simulink library "bcm"  (R2021b)
settings: Solver=VariableStepAuto  StartTime=0.0  StopTime=10.0  RelTol=1e-3
undefined symbols (not defined in the file or in its folder): ENUM_ANTITHEFT_ALARM, ENUM_ANTITHEFT_ARM, ENUM_ANTITHEFT_DISARM, ENUM_ANTITHEFT_WAIT, ENUM_GEARPOSNTOCAN_P, ENUM_PDKEYRAWLULOCK_INUNLOCK, ENUM_PDKEYRAWPS_INPS, ENUM_POWERSTA_ON, ENUM_POWERSTA_READY, ENUM_POWERSTA_STANDBY, ENUM_PWRSTASW_ON, ENUM_PWRSTASW_READY, ENUM_VEHICLETYPE_D21, ENUM_VEHICLETYPE_D31F25, ENUM_VEHICLETYPE_D31HAWD, ENUM_VEHICLETYPE_D31HRWD, ENUM_VEHICLETYPE_D31L24, FALSE, KBCM_ACCSwcPrsTmr_s, KBCM_ALMBrightnessDark_enum, KBCM_AmbBlue_enum, KBCM_AmbBreathT_ms, KBCM_AmbGreen_enum, KBCM_AmbMidPple_enum, KBCM_AmbRed_enum, KBCM_AmbTempCtrlEN_flg, KBCM_AmbTempT_s, KBCM_AmbWelModeENWait_s, KBCM_Antitheft_enum_ovrdflg, KBCM_Antitheft_enum_ovrdval, KBCM_APMDoorCtrlSta_flg_ovrdflg, KBCM_APMDoorCtrlSta_flg_ovrdval, KBCM_CmdKeepT_s, KBCM_CSWLightRstDebT_s, KBCM_CSWTurnLPRstT_s, KBCM_DelayTSW_flg, KBCM_DiagDRLOFF_flg, KBCM_DiagFLTC_mA, KBCM_DiagFMHT_s, KBCM_DiagFRTC_mA, KBCM_DiagRLTC_mA, KBCM_DiagRRTC_mA, KBCM_DrAPMRetryTimes_cnt, KBCM_DrOpenWdwOT_s, KBCM_DrOpenWdwReady_s, KBCM_ESSOffT_ms, KBCM_ESSOnT_ms, KBCM_FDCDKCReDetectT_K, KBCM_FDCDKCUSSFilterT_K, KBCM_HandleLampKeepT_s, KBCM_IVIRstHoldT_ms, KBCM_IVIRstTriggerT_ms, KBCM_ONDelayT_ms, KBCM_RAPSAbnFlashOFFT_ms, KBCM_RAPSAbnFlashONT_ms, KBCM_ReDetectT_K, KBCM_RightHandDriveEN_flg, KBCM_RLSLowSpdFilterT_s, KBCM_RmLampKeep_min, KBCM_RmLpKeyInT_s ... (+37)
libraries: simulink x389, $bdroot x11, hcu_lib x2
(part 5 of 13)

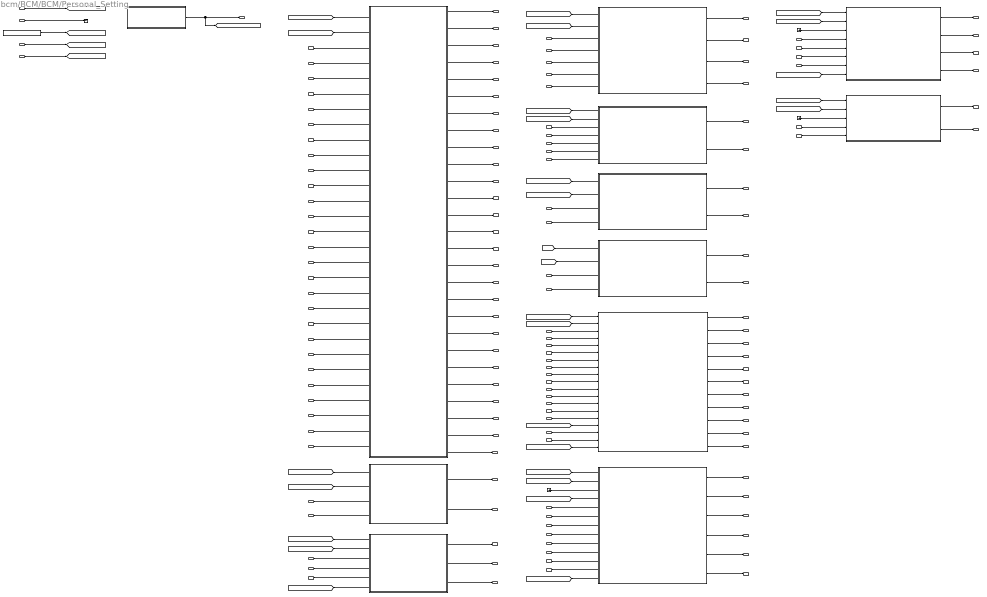
== system bcm/BCM/BCM/Personal_Setting ==
  task_time_s : Inport
  UserNow : Inport  Port=2
  VINP_CANMsgValidIVI1_flg : Inport  Port=3
  VINP_AmbLightSW_flg : Inport  Port=4
  VINP_FlashAmbFunEN_enum : Inport  Port=5
  VINP_AmbLightWlcmLightSW_flg : Inport  Port=6
  VINP_FlashAmbWelEN_enum : Inport  Port=7
  VINP_AmbLightDimInDarkSW_flg : Inport  Port=8
  VINP_FlashAmbDimEN_enum : Inport  Port=9
  VINP_LINKtoDRIVE_flg : Inport  Port=10
  VINP_FlashAmbLinkDriSta_enum : Inport  Port=11
  VINP_AmbLighLowBatAlertSW_flg : Inport  Port=12
  VINP_FlashAmbPwrWarnEN_enum : Inport  Port=13
  VINP_AmbLighSafetyAlertSW_flg : Inport  Port=14
  VINP_FlashAmbODAEN_enum : Inport  Port=15
  VINP_AmbLightColorSet_enum : Inport  Port=16
  VINP_FlashAmbColorSta1_enum : Inport  Port=17
  VINP_FlashAmbColorSta2_enum : Inport  Port=18
  VINP_FlashAmbColorSta3_enum : Inport  Port=19
  VINP_FlashAmbColorSta4_enum : Inport  Port=20
  VINP_FlashAmbColorSta5_enum : Inport  Port=21
  VINP_FlashAmbColorSta7_enum : Inport  Port=22
  VINP_AmbLightBrightnessSet_enum : Inport  Port=23
  VINP_FlashAmbBrightnessSta1_enum : Inport  Port=24
  VINP_FlashAmbBrightnessSta2_enum : Inport  Port=25
  VINP_FlashAmbBrightnessSta3_enum : Inport  Port=26
  VINP_FlashAmbBrightnessSta4_enum : Inport  Port=27
  VINP_FlashAmbBrightnessSta5_enum : Inport  Port=28
  VINP_FlashAmbBrightnessSta7_enum : Inport  Port=29
  VINP_IVIPTGUSStaSW_flg : Inport  Port=30
  VINP_FlashSPTGENFun_enum : Inport  Port=31
  VINP_TurnSwTimeSet_enum : Inport  Port=32
  VINP_FlashTurnSwTimeSetSta123_enum : Inport  Port=33
  VINP_FlashTurnSwTimeSetSta457_enum : Inport  Port=34
  VINP_CANMsgValidIVI2_flg : Inport  Port=35
  VINP_ApproachUnlockSW_flg : Inport  Port=36
  VINP_FlashWalkInUnLkEn_enum : Inport  Port=37
  VINP_WalkawayLockSW_flg : Inport  Port=38
  VINP_FlashWalkOutLkEn_enum : Inport  Port=39
  VINP_RoomLampMode_flg : Inport  Port=40
  VINP_FlashRmLpModeEN_enum : Inport  Port=41
  VINP_SetUnlockSingle_flg : Inport  Port=42
  VINP_FlashLockSettingSta_enum : Inport  Port=43
  VINP_FollowMeSW_flg : Inport  Port=44
  VINP_FlashFollowMeENFun_enum : Inport  Port=45
  VINP_IVIPTGOpenHeight_enum : Inport  Port=46
  VINP_FlashPTGOpenHeight12_enum : Inport  Port=47
  VINP_FlashPTGOpenHeight34_enum : Inport  Port=48
  VINP_FlashPTGOpenHeight57_enum : Inport  Port=49
  VINP_PTGIsSetHeight_flg : Inport  Port=50
  VINP_BPPTGIsSetHeightSta_flg : Inport  Port=51
  VINP_PTGLeftHallPosn_cnt : Inport  Port=52
  VINP_FlashPTGUserHeight1_cnt : Inport  Port=53
  VINP_FlashPTGUserHeight2_cnt : Inport  Port=54
  VINP_FlashPTGUserHeight3_cnt : Inport  Port=55
  VINP_FlashPTGUserHeight4_cnt : Inport  Port=56
  VINP_FlashPTGUserHeight5_cnt : Inport  Port=57
  VINP_FlashPTGUserHeight7_cnt : Inport  Port=58
  VINP_TimeGapLevel_enum : Inport  Port=59
  VINP_FlashACCLevelSta12_enum : Inport  Port=60
  VINP_FlashACCLevelSta34_enum : Inport  Port=61
  VINP_FlashACCLevelSta57_enum : Inport  Port=62
  VINP_SWC2LRightSta_flg : Inport  Port=63
  VINP_SWC2LLeftSta_flg : Inport  Port=64
  VINP_FDCVMCSpdCtrlModeSta_enum : Inport  Port=65
  VINP_ADASACCSta_enum : Inport  Port=66
  VINP_IVIStoppingUnlockSWSta_flg : Inport  Port=67
  VINP_FlashAutoLock_enum : Inport  Port=68
  VINP_IVIDrivingLockSWSta_flg : Inport  Port=69
  VINP_FlashAutoUnlock_enum : Inport  Port=70
  VINP_CANMsgValidBodyZonePS1_flg : Inport  Port=71
  VINP_LeftHallPos_cnt : Inport  Port=72
  VINP_VehicleType_enum : Inport  Port=73
  VINP_SWC2RCustomizeSta_flg : Inport  Port=74
  VINP_IVISWCRUndefinedSta_enum : Inport  Port=75
  VINP_HMIAutoInterLightCmd_flg : Inport  Port=76
  VINP_IVICLWinLockDrSW_flg : Inport  Port=77
  VINP_FlashCLWinLockDrSta_enum : Inport  Port=78
  VINP_IVICarWashModeCmd_flg : Inport  Port=79
  ACC : Subsystem
  AmbLight : Subsystem
  Autolock : Subsystem
  Constant : Constant  Value=KBCM_UserFix_enum
  DKC_Lock_Setting : Subsystem
  FlasherSignal : Subsystem
  FollowMeHome : Subsystem
  Ground : Ground
  Ground1 : Ground
  Ground4 : Ground
  LockSetting : Subsystem
  PTG : Subsystem
  RoomLamp : Subsystem
  SPTG : Subsystem
  System_Loadbar : Subsystem
  Terminator : Terminator
  Window : Subsystem
  Loadbar : Outport
  VBCM_UserNow_enum : Outport  Port=2
  FDC_BCM_AmbFunEN_Sta : Outport  Port=3
  VBCM_AmbFunENMem_enum : Outport  Port=4
  FDC_BCM_AmbWelEN_Sta : Outport  Port=5
  VBCM_AmbWelENMem_enum : Outport  Port=6
  FDC_BCM_AmbDimEN_Sta : Outport  Port=7
  VBCM_AmbDimENMem_enum : Outport  Port=8
  FDC_BCM_AmbLinkDriSta_Sta : Outport  Port=9
  VBCM_AmbLinkDriStaMem_enum : Outport  Port=10
  FDC_BCM_AmbPwrWarnEN_Sta : Outport  Port=11
  VBCM_AmbPwrWarnENMem_enum : Outport  Port=12
  FDC_BCM_AmbODAEN_Sta : Outport  Port=13
  VBCM_AmbODAENMem_enum : Outport  Port=14
  FDC_BCM_AmbColorSta_Sta : Outport  Port=15
  VBCM_AmbColorSta1_enum : Outport  Port=16
  VBCM_AmbColorSta2_enum : Outport  Port=17
  VBCM_AmbColorSta3_enum : Outport  Port=18
  VBCM_AmbColorSta4_enum : Outport  Port=19
  VBCM_AmbColorSta5_enum : Outport  Port=20
  VBCM_AmbColorSta7_enum : Outport  Port=21
  FDC_BCM_AmbBrightSta_Sta : Outport  Port=22
  VBCM_AmbBrightnessSta1_enum : Outport  Port=23
  VBCM_AmbBrightnessSta2_enum : Outport  Port=24
  VBCM_AmbBrightnessSta3_enum : Outport  Port=25
  VBCM_AmbBrightnessSta4_enum : Outport  Port=26
  VBCM_AmbBrightnessSta5_enum : Outport  Port=27
  VBCM_AmbBrightnessSta7_enum : Outport  Port=28
  VBCM_SPTGENFun_flg : Outport  Port=29
  VBCM_SPTGENFunMem_enum : Outport  Port=30
  VBCM_TurnSwTSetSta_enum : Outport  Port=31
  VBCM_TurnSwTimeSetSta123_enum : Outport  Port=32
  VBCM_TurnSwTimeSetSta457_enum : Outport  Port=33
  FDC_BCM_WalkInUnLkEnFun_Sta : Outport  Port=34
  VBCM_WalkInUnLkEnMem_enum : Outport  Port=35
  FDC_BCM_WalkOutLkEnFun_Sta : Outport  Port=36
  VBCM_WalkOutLkEnMem_enum : Outport  Port=37
  FDC_BCM_RmLpModeENFun_Sta : Outport  Port=38
  VBCM_RmLpModeENMem_enum : Outport  Port=39
  VBCM_LockSetting_flg : Outport  Port=40
  VBCM_LockSettingStaMem_enum : Outport  Port=41
  FDC_BCM_FollowMeENFun_Sta : Outport  Port=42
  VBCM_FollowMeENMem_enum : Outport  Port=43
  VBCM_PTGOpenHeightSta_enum : Outport  Port=44
  VBCM_UserHeightSet_cnt : Outport  Port=45
  VBCM_PTGUserHeight1_cnt : Outport  Port=46
  VBCM_PTGUserHeight2_cnt : Outport  Port=47
  VBCM_PTGUserHeight3_cnt : Outport  Port=48
  VBCM_PTGUserHeight4_cnt : Outport  Port=49
  VBCM_PTGUserHeight5_cnt : Outport  Port=50
  VBCM_PTGUserHeight7_cnt : Outport  Port=51
  VBCM_PTGOpenHeight12_enum : Outport  Port=52
  VBCM_PTGOpenHeight34_enum : Outport  Port=53
  VBCM_PTGOpenHeight57_enum : Outport  Port=54
  VBCM_TimeGapLevelSta_enum : Outport  Port=55
  VBCM_ACCLevelMem12_enum : Outport  Port=56
  VBCM_ACCLevelMem34_enum : Outport  Port=57
  VBCM_ACCLevelMem57_enum : Outport  Port=58
  VBCM_LRightStaCmd_flg : Outport  Port=59
  VBCM_LLeftStaCmd_flg : Outport  Port=60
  VBCM_AutoLockSta_flg : Outport  Port=61
  VBCM_AutoLockMem_enum : Outport  Port=62
  VBCM_AutoUnlockSta_flg : Outport  Port=63
  VBCM_AutoUnlockMem_enum : Outport  Port=64
  VBCM_CLWinLockDrSta_flg : Outport  Port=65
  VBCM_CLWinLockDrStaMem_enum : Outport  Port=66
  wires:
  VINP_FlashAmbFunEN_enum/1 -> AmbLight/5(VINP_FlashAmbFunEN_enum)
  VINP_FlashAmbBrightnessSta3_enum/1 -> AmbLight/26(VINP_FlashAmbBrightnessSta3_enum)
  VINP_FlashAmbBrightnessSta7_enum/1 -> AmbLight/29(VINP_FlashAmbBrightnessSta7_enum)
  VINP_FlashAmbColorSta7_enum/1 -> AmbLight/22(VINP_FlashAmbColorSta7_enum)
  VINP_FlashAmbColorSta5_enum/1 -> AmbLight/21(VINP_FlashAmbColorSta5_enum)
  VINP_FlashAmbColorSta1_enum/1 -> AmbLight/17(VINP_FlashAmbColorSta1_enum)
  VINP_FlashAmbDimEN_enum/1 -> AmbLight/9(VINP_FlashAmbDimEN_enum)
  VINP_AmbLightSW_flg/1 -> AmbLight/4(VINP_AmbLightSW_flg)
  VINP_FlashAmbColorSta3_enum/1 -> AmbLight/19(VINP_FlashAmbColorSta3_enum)
  VINP_FlashAmbColorSta4_enum/1 -> AmbLight/20(VINP_FlashAmbColorSta4_enum)
  VINP_FlashAmbODAEN_enum/1 -> AmbLight/15(VINP_FlashAmbODAEN_enum)
  VINP_AmbLightWlcmLightSW_flg/1 -> AmbLight/6(VINP_AmbLightWlcmLightSW_flg)
  AmbLight/4(FDC_BCM_AmbWelEN_Sta) -> FDC_BCM_AmbWelEN_Sta/1
  VINP_AmbLighLowBatAlertSW_flg/1 -> AmbLight/12(VINP_AmbLighLowBatAlertSW_flg)
  AmbLight/14(FDC_BCM_AmbColorSta_Sta) -> FDC_BCM_AmbColorSta_Sta/1
  AmbLight/10(FDC_BCM_AmbPwrWarnEN_Sta) -> FDC_BCM_AmbPwrWarnEN_Sta/1
  VINP_AmbLightBrightnessSet_enum/1 -> AmbLight/23(VINP_AmbLightBrightnessSet_enum)
  VINP_AmbLighSafetyAlertSW_flg/1 -> AmbLight/14(VINP_AmbLighSafetyAlertSW_flg)
  AmbLight/2(FDC_BCM_AmbFunEN_Sta) -> FDC_BCM_AmbFunEN_Sta/1
  AmbLight/6(FDC_BCM_AmbDimEN_Sta) -> FDC_BCM_AmbDimEN_Sta/1
  AmbLight/8(FDC_BCM_AmbLinkDriSta_Sta) -> FDC_BCM_AmbLinkDriSta_Sta/1
  VINP_LINKtoDRIVE_flg/1 -> AmbLight/10(VINP_LINKtoDRIVE_flg)
  VINP_FlashAmbBrightnessSta2_enum/1 -> AmbLight/25(VINP_FlashAmbBrightnessSta2_enum)
  VINP_FlashAmbColorSta2_enum/1 -> AmbLight/18(VINP_FlashAmbColorSta2_enum)
  VINP_AmbLightDimInDarkSW_flg/1 -> AmbLight/8(VINP_AmbLightDimInDarkSW_flg)
  VINP_FlashAmbLinkDriSta_enum/1 -> AmbLight/11(VINP_FlashAmbLinkDriSta_enum)
  VINP_AmbLightColorSet_enum/1 -> AmbLight/16(VINP_AmbLightColorSet_enum)
  VINP_FlashAmbBrightnessSta4_enum/1 -> AmbLight/27(VINP_FlashAmbBrightnessSta4_enum)
  VINP_FlashAmbPwrWarnEN_enum/1 -> AmbLight/13(VINP_FlashAmbPwrWarnEN_enum)
  [Loadbar] -> AmbLight/2(Loadbar)
  VINP_FlashAmbBrightnessSta5_enum/1 -> AmbLight/28(VINP_FlashAmbBrightnessSta5_enum)
  VINP_FlashAmbBrightnessSta1_enum/1 -> AmbLight/24(VINP_FlashAmbBrightnessSta1_enum)
  AmbLight/21(FDC_BCM_AmbBrightSta_Sta) -> FDC_BCM_AmbBrightSta_Sta/1
  AmbLight/12(FDC_BCM_AmbODAEN_Sta) -> FDC_BCM_AmbODAEN_Sta/1
  VINP_FlashAmbWelEN_enum/1 -> AmbLight/7(VINP_FlashAmbWelEN_enum)
  System_Loadbar/1(Loadbar) -> [Loadbar], Loadbar/1
  AmbLight/3(VBCM_AmbFunENMem_enum) -> VBCM_AmbFunENMem_enum/1
  AmbLight/5(VBCM_AmbWelENMem_enum) -> VBCM_AmbWelENMem_enum/1
  AmbLight/7(VBCM_AmbDimENMem_enum) -> VBCM_AmbDimENMem_enum/1
  AmbLight/9(VBCM_AmbLinkDriStaMem_enum) -> VBCM_AmbLinkDriStaMem_enum/1
  AmbLight/11(VBCM_AmbPwrWarnENMem_enum) -> VBCM_AmbPwrWarnENMem_enum/1
  AmbLight/13(VBCM_AmbODAENMem_enum) -> VBCM_AmbODAENMem_enum/1
  AmbLight/15(VBCM_AmbColorSta1_enum) -> VBCM_AmbColorSta1_enum/1
  AmbLight/16(VBCM_AmbColorSta2_enum) -> VBCM_AmbColorSta2_enum/1
  AmbLight/17(VBCM_AmbColorSta3_enum) -> VBCM_AmbColorSta3_enum/1
  AmbLight/18(VBCM_AmbColorSta4_enum) -> VBCM_AmbColorSta4_enum/1
  AmbLight/19(VBCM_AmbColorSta5_enum) -> VBCM_AmbColorSta5_enum/1
  AmbLight/20(VBCM_AmbColorSta7_enum) -> VBCM_AmbColorSta7_enum/1
  AmbLight/22(VBCM_AmbBrightnessSta1_enum) -> VBCM_AmbBrightnessSta1_enum/1
  AmbLight/23(VBCM_AmbBrightnessSta2_enum) -> VBCM_AmbBrightnessSta2_enum/1
  AmbLight/24(VBCM_AmbBrightnessSta3_enum) -> VBCM_AmbBrightnessSta3_enum/1
  AmbLight/25(VBCM_AmbBrightnessSta4_enum) -> VBCM_AmbBrightnessSta4_enum/1
  AmbLight/26(VBCM_AmbBrightnessSta5_enum) -> VBCM_AmbBrightnessSta5_enum/1
  AmbLight/27(VBCM_AmbBrightnessSta7_enum) -> VBCM_AmbBrightnessSta7_enum/1
  VINP_CANMsgValidIVI1_flg/1 -> AmbLight/3(VINP_CANMsgValidIVI1_flg)
  AmbLight/1(VBCM_UserNow_enum) -> VBCM_UserNow_enum/1
  SPTG/1(FDC_SPTG_SPTGENFun_Sta) -> VBCM_SPTGENFun_flg/1  "VBCM_SPTGENFun_flg"
  SPTG/2(VBCM_SPTGENFunMem_enum) -> VBCM_SPTGENFunMem_enum/1  "VBCM_SPTGENFunMem_enum"
  [UserNow] -> AmbLight/1(UserNow)
  [UserNow] -> SPTG/1(UserNow)
  UserNow/1 -> Terminator/1
  [Loadbar] -> SPTG/2(Loadbar)
  VINP_IVIPTGUSStaSW_flg/1 -> SPTG/3(VINP_IVIPTGUSStaSW_flg)
  VINP_FlashSPTGENFun_enum/1 -> SPTG/4(VINP_FlashSPTGENFun_enum)
  [UserNow] -> FlasherSignal/1(UserNow)
  [Loadbar] -> FlasherSignal/2(Loadbar)
  FlasherSignal/1(FDC_BCM_TurnSwTSetSta_Sta) -> VBCM_TurnSwTSetSta_enum/1  "FDC_BCM_TurnSwTSetSta_Sta"
  FlasherSignal/2(VBCM_TurnSwTimeSetSta123_enum) -> VBCM_TurnSwTimeSetSta123_enum/1  "VBCM_TurnSwTimeSetSta123_enum"
  FlasherSignal/3(VBCM_TurnSwTimeSetSta457_enum) -> VBCM_TurnSwTimeSetSta457_enum/1  "VBCM_TurnSwTimeSetSta457_enum"
  VINP_TurnSwTimeSet_enum/1 -> FlasherSignal/3(VINP_TurnSwTimeSet_enum)
  VINP_FlashTurnSwTimeSetSta457_enum/1 -> FlasherSignal/5(VINP_FlashTurnSwTimeSetSta457_enum)
  VINP_FlashTurnSwTimeSetSta123_enum/1 -> FlasherSignal/4(VINP_FlashTurnSwTimeSetSta123_enum)
  Constant/1 -> [UserNow]
  [Loadbar] -> DKC_Lock_Setting/2(Loadbar)
  [UserNow] -> DKC_Lock_Setting/1(UserNow)
  VINP_ApproachUnlockSW_flg/1 -> DKC_Lock_Setting/3(VINP_ApproachUnlockSW_flg)
  VINP_FlashWalkInUnLkEn_enum/1 -> DKC_Lock_Setting/4(VINP_FlashWalkInUnLkEn_enum)
  VINP_WalkawayLockSW_flg/1 -> DKC_Lock_Setting/6(VINP_WalkawayLockSW_flg)
  VINP_FlashWalkOutLkEn_enum/1 -> DKC_Lock_Setting/7(VINP_FlashWalkOutLkEn_enum)
  DKC_Lock_Setting/1(FDC_BCM_WalkInUnLkEnFun_Sta) -> FDC_BCM_WalkInUnLkEnFun_Sta/1
  DKC_Lock_Setting/2(VBCM_WalkInUnLkEnMem_enum) -> VBCM_WalkInUnLkEnMem_enum/1
  DKC_Lock_Setting/3(FDC_BCM_WalkOutLkEnFun_Sta) -> FDC_BCM_WalkOutLkEnFun_Sta/1
  DKC_Lock_Setting/4(VBCM_WalkOutLkEnMem_enum) -> VBCM_WalkOutLkEnMem_enum/1
  [Loadbar] -> RoomLamp/2(Loadbar)
  [UserNow] -> RoomLamp/1(UserNow)
  VINP_RoomLampMode_flg/1 -> RoomLamp/3(VINP_RoomLampMode_flg)
  VINP_FlashRmLpModeEN_enum/1 -> RoomLamp/4(VINP_FlashRmLpModeEN_enum)
  RoomLamp/1(FDC_BCM_RmLpModeENFun_Sta) -> FDC_BCM_RmLpModeENFun_Sta/1
  RoomLamp/2(VBCM_RmLpModeENMem_enum) -> VBCM_RmLpModeENMem_enum/1
  LockSetting/2(VBCM_LockSettingStaMem_enum) -> VBCM_LockSettingStaMem_enum/1
  LockSetting/1(VBCM_LockSetting_flg) -> VBCM_LockSetting_flg/1
  VINP_FlashLockSettingSta_enum/1 -> LockSetting/4(VINP_FlashLockSettingSta_enum)
  VINP_SetUnlockSingle_flg/1 -> LockSetting/3(VINP_SetUnlockSingle_flg)
  [UserNow] -> LockSetting/1(UserNow)
  [Loadbar] -> LockSetting/2(Loadbar)
  [Loadbar] -> FollowMeHome/2(Loadbar)
  [UserNow] -> FollowMeHome/1(UserNow)
  VINP_FollowMeSW_flg/1 -> FollowMeHome/3(VINP_FollowMeSW_flg)
  VINP_FlashFollowMeENFun_enum/1 -> FollowMeHome/4(VINP_FlashFollowMeENFun_enum)
  FollowMeHome/1(FDC_BCM_FollowMeENFun_Sta) -> FDC_BCM_FollowMeENFun_Sta/1
  FollowMeHome/2(VBCM_FollowMeENMem_enum) -> VBCM_FollowMeENMem_enum/1
  PTG/2(VBCM_UserHeightSet_cnt) -> VBCM_UserHeightSet_cnt/1
  PTG/1(VBCM_PTGOpenHeightSta_enum) -> VBCM_PTGOpenHeightSta_enum/1
  PTG/7(VBCM_PTGUserHeight5_cnt) -> VBCM_PTGUserHeight5_cnt/1
  PTG/8(VBCM_PTGUserHeight7_cnt) -> VBCM_PTGUserHeight7_cnt/1
  PTG/4(VBCM_PTGUserHeight2_cnt) -> VBCM_PTGUserHeight2_cnt/1
  PTG/5(VBCM_PTGUserHeight3_cnt) -> VBCM_PTGUserHeight3_cnt/1
  PTG/6(VBCM_PTGUserHeight4_cnt) -> VBCM_PTGUserHeight4_cnt/1
  PTG/3(VBCM_PTGUserHeight1_cnt) -> VBCM_PTGUserHeight1_cnt/1
  VINP_CANMsgValidIVI2_flg/1 -> [VINP_CANMsgValidIVI2_flg]
  [VINP_CANMsgValidIVI2_flg] -> FlasherSignal/6(VINP_CANMsgValidIVI2_flg)
  [VINP_CANMsgValidIVI2_flg] -> PTG/16(VINP_CANMsgValidIVI2_flg)
  [Loadbar] -> PTG/2(Loadbar)
  [UserNow] -> PTG/1(UserNow)
  VINP_IVIPTGOpenHeight_enum/1 -> PTG/3(VINP_IVIPTGOpenHeight_enum)
  VINP_FlashPTGOpenHeight12_enum/1 -> PTG/4(VINP_FlashPTGOpenHeight12_enum)
  VINP_BPPTGIsSetHeightSta_flg/1 -> PTG/8(VINP_BPPTGIsSetHeightSta_flg)
  VINP_FlashPTGOpenHeight34_enum/1 -> PTG/5(VINP_FlashPTGOpenHeight34_enum)
  VINP_FlashPTGOpenHeight57_enum/1 -> PTG/6(VINP_FlashPTGOpenHeight57_enum)
  VINP_PTGLeftHallPosn_cnt/1 -> PTG/9(VINP_PTGLeftHallPosn_cnt)
  VINP_FlashPTGUserHeight1_cnt/1 -> PTG/10(VINP_FlashPTGUserHeight1_cnt)
  VINP_FlashPTGUserHeight2_cnt/1 -> PTG/11(VINP_FlashPTGUserHeight2_cnt)
  VINP_FlashPTGUserHeight3_cnt/1 -> PTG/12(VINP_FlashPTGUserHeight3_cnt)
  VINP_FlashPTGUserHeight4_cnt/1 -> PTG/13(VINP_FlashPTGUserHeight4_cnt)
  VINP_FlashPTGUserHeight5_cnt/1 -> PTG/14(VINP_FlashPTGUserHeight5_cnt)
  VINP_FlashPTGUserHeight7_cnt/1 -> PTG/15(VINP_FlashPTGUserHeight7_cnt)
  PTG/9(VBCM_PTGOpenHeight12_enum) -> VBCM_PTGOpenHeight12_enum/1
  PTG/10(VBCM_PTGOpenHeight34_enum) -> VBCM_PTGOpenHeight34_enum/1
  PTG/11(VBCM_PTGOpenHeight57_enum) -> VBCM_PTGOpenHeight57_enum/1
  VINP_PTGIsSetHeight_flg/1 -> PTG/7(VINP_PTGIsSetHeight_flg)
  VINP_SWC2LRightSta_flg/1 -> ACC/9(VINP_SWC2LRightSta_flg)
  ACC/3(VBCM_ACCLevelMem34_enum) -> VBCM_ACCLevelMem34_enum/1
  ACC/4(VBCM_ACCLevelMem57_enum) -> VBCM_ACCLevelMem57_enum/1
  [UserNow] -> ACC/1(UserNow)
  ACC/5(VBCM_LRightStaCmd_flg) -> VBCM_LRightStaCmd_flg/1
  VINP_FDCVMCSpdCtrlModeSta_enum/1 -> ACC/11(VINP_FDCVMCSpdCtrlModeSta_enum)
  ACC/1(VBCM_TimeGapLevelSta_enum) -> VBCM_TimeGapLevelSta_enum/1
  VINP_ADASACCSta_enum/1 -> ACC/12(VINP_ADASACCSta_enum)
  ACC/6(VBCM_LLeftStaCmd_flg) -> VBCM_LLeftStaCmd_flg/1
  ACC/2(VBCM_ACCLevelMem12_enum) -> VBCM_ACCLevelMem12_enum/1
  VINP_FlashACCLevelSta12_enum/1 -> ACC/6(VINP_FlashACCLevelSta12_enum)
  VINP_SWC2LLeftSta_flg/1 -> ACC/10(VINP_SWC2LLeftSta_flg)
  VINP_FlashACCLevelSta57_enum/1 -> ACC/8(VINP_FlashACCLevelSta57_enum)
  VINP_FlashACCLevelSta34_enum/1 -> ACC/7(VINP_FlashACCLevelSta34_enum)
  [task_time_s] -> ACC/4(task_time_s)
  VINP_TimeGapLevel_enum/1 -> ACC/5(VINP_TimeGapLevel_enum)
  Ground/1 -> ACC/3(UpdateReq)
  [Loadbar] -> ACC/2(Loadbar)
  task_time_s/1 -> [task_time_s]
  VINP_IVIStoppingUnlockSWSta_flg/1 -> Autolock/4(VINP_IVIStoppingUnlockSWSta_flg)
  Autolock/3(VBCM_AutoUnlockSta_flg) -> VBCM_AutoUnlockSta_flg/1
  Autolock/4(VBCM_AutoUnlockMem_enum) -> VBCM_AutoUnlockMem_enum/1
  Ground1/1 -> Autolock/3(VBCM_SettingUpdateReq_enum)
  Autolock/2(VBCM_AutoLockMem_enum) -> VBCM_AutoLockMem_enum/1
  VINP_FlashAutoUnlock_enum/1 -> Autolock/7(VINP_FlashAutoUnlock_enum)
  Autolock/1(VBCM_AutoLockSta_flg) -> VBCM_AutoLockSta_flg/1
  VINP_IVIDrivingLockSWSta_flg/1 -> Autolock/6(VINP_IVIDrivingLockSWSta_flg)
  [UserNow] -> Autolock/1(UserNow)
  VINP_FlashAutoLock_enum/1 -> Autolock/5(VINP_FlashAutoLock_enum)
  [Loadbar] -> Autolock/2(Loadbar)
  VINP_CANMsgValidBodyZonePS1_flg/1 -> PTG/17(VINP_CANMsgValidBodyZonePS1_flg)
  VINP_LeftHallPos_cnt/1 -> PTG/18(VINP_LeftHallPos_cnt)
  VINP_VehicleType_enum/1 -> [VINP_VehicleType_enum]
  [VINP_VehicleType_enum] -> ACC/13(VINP_VehicleType_enum)
  [VINP_VehicleType_enum] -> PTG/19(VINP_VehicleType_enum)
  [VINP_VehicleType_enum] -> Autolock/8(VINP_VehicleType_enum)
  VINP_SWC2RCustomizeSta_flg/1 -> RoomLamp/5(VINP_SWC2RCustomizeSta_flg)
  VINP_IVISWCRUndefinedSta_enum/1 -> RoomLamp/6(VINP_IVISWCRUndefinedSta_enum)
  VINP_HMIAutoInterLightCmd_flg/1 -> RoomLamp/7(HMI_AutoInterLight_Cmd)
  Window/1(VBCM_CLWinLockDrSta_flg) -> VBCM_CLWinLockDrSta_flg/1
  Window/2(VBCM_CLWinLockDrStaMem_enum) -> VBCM_CLWinLockDrStaMem_enum/1
  [Loadbar] -> Window/2(Loadbar)
  [UserNow] -> Window/1(UserNow)
  VINP_IVICLWinLockDrSW_flg/1 -> Window/4(VINP_IVICLWinLockDrSW_flg)
  VINP_FlashCLWinLockDrSta_enum/1 -> Window/5(VINP_FlashCLWinLockDrSta_enum)
  Ground4/1 -> Window/3(UpdateReq)
  VINP_IVICarWashModeCmd_flg/1 -> DKC_Lock_Setting/5(VINP_IVICarWashModeCmd_flg)

== system bcm/BCM/BCM/PowerMirror ==
  VPMM_PwrSta_enum : Inport
  VINP_MIRRORFOLDSW_flg : Inport  Port=2
  VINP_VehSpeed_kph : Inport  Port=3
  VBCM_ATActCtrl_enum : Inport  Port=4
  VINP_ReOutsideMirror_enum : Inport  Port=5
  EEP_MFSWTri_flg : Inport  Port=6
  EEP_MirrorFlodPos : Inport  Port=7
  VINP_APSStaSystem_enum : Inport  Port=8
  VINP_IVICarWashModeCmd_flg : Inport  Port=9
  VINP_IVIMirrorFoldedSWSta_flg : Inport  Port=10
  VINP_DKCParkingModeCmd_enum : Inport  Port=11
  AND : Logic  AllPortsSameDT=off  OutDataTypeStr=boolean
  Chart : Stateflow chart  TreatAsAtomicUnit=on
  Compare To Constant : simulink/Logic and Bit Operations/Compare To Constant  relop===  const=0  OutDataTypeStr=boolean
  Compare To Constant1 : simulink/Logic and Bit Operations/Compare To Constant  relop===  const=1  OutDataTypeStr=boolean
  Detect Increase : simulink/Logic and Bit Operations/Detect Increase  vinit=0.0  OutDataTypeStr=boolean
  Unit Delay : UnitDelay  SampleTime=-1  HasFrameUpgradeWarning=on
  VBCM_MirrorCtrl_enum : Outport
  MFSWTri : Outport  Port=2
  MirrorFlodPos : Outport  Port=3
  wires:
  VPMM_PwrSta_enum/1 -> Chart/1(PwrSta)
  VINP_MIRRORFOLDSW_flg/1 -> Chart/2(MirrorFoldSw)
  Chart/1(MirrorCtrl) -> VBCM_MirrorCtrl_enum/1  "VBCM_MirrorCtrl_enum"
  VBCM_ATActCtrl_enum/1 -> Chart/4(ATActCtrl)
  VINP_VehSpeed_kph/1 -> Chart/3(VehSpeed)
  VINP_ReOutsideMirror_enum/1 -> Chart/5(VINP_ReOutsideMirror_enum)
  EEP_MFSWTri_flg/1 -> Chart/6(EEP_MFSWTri_flg)
  EEP_MirrorFlodPos/1 -> Chart/7(EEP_MirrorFlodPos)
  Chart/2(MFSWTri) -> MFSWTri/1  "VBCM_MFSWTri_flg"
  Chart/3(MirrorFlodPos) -> MirrorFlodPos/1  "VBCM_MirrorFlodPos_flg"
  VINP_APSStaSystem_enum/1 -> Chart/8(APS_Sta_System)
  VINP_IVICarWashModeCmd_flg/1 -> Chart/9(IVICarWashModeCmd)
  VINP_IVIMirrorFoldedSWSta_flg/1 -> Detect Increase/1
  Detect Increase/1 -> Chart/10(IVIMirrorFoldedReq)
  AND/1 -> Chart/11(VBCM_RAPSActivate_flg)
  Compare To Constant/1 -> AND/1
  Compare To Constant1/1 -> AND/2
  Unit Delay/1 -> Compare To Constant/1
  VINP_DKCParkingModeCmd_enum/1 -> Compare To Constant1/1, Unit Delay/1

== system bcm/BCM/BCM/RearDefogger ==
  VPMM_PwrSta_enum : Inport
  VINP_RRDefSta_flg : Inport  Port=2
  VINP_IVIRRDefReq_flg : Inport  Port=3
  Chart : Stateflow chart  TreatAsAtomicUnit=on
  VBCM_MirrorDefog_flg : Outport
  VBCM_RrDefog_flg : Outport  Port=2
  wires:
  Chart/1(MirrorDefog) -> VBCM_MirrorDefog_flg/1  "VBCM_MirrorDefog_flg"
  VINP_IVIRRDefReq_flg/1 -> Chart/3(IVI_RR_Def_Req)
  VPMM_PwrSta_enum/1 -> Chart/1(PwrSta)
  Chart/2(RearDefog) -> VBCM_RrDefog_flg/1  "VBCM_RrDefog_flg"
  VINP_RRDefSta_flg/1 -> Chart/2(RR_Def_Sta)

== system bcm/BCM/BCM/RoomLamp ==
  task_time_s : Inport
  VPMM_PwrSta_enum : Inport  Port=2
  VBCM_BCMDoorLockSta_flg : Inport  Port=3
  VBCM_AllDoorSW_flg : Inport  Port=4
  VBCM_AntitheftSta_enum : Inport  Port=5
  VINP_DrDoorSW_flg : Inport  Port=6
  VINP_PsDoorSW_flg : Inport  Port=7
  VINP_RLDoorSW_flg : Inport  Port=8
  VINP_RRDoorSW_flg : Inport  Port=9
  FDC_BCM_RmLpModeENFun_Sta : Inport  Port=10
  VINP_TailgateSW_flg : Inport  Port=11
  KBCM_RmLampKeep_min : Inport  Port=12
  VINP_PDKeyAreaLockUnlock_enum : Inport  Port=13
  VINP_PDKeyAreaPS_enum : Inport  Port=14
  KBCM_RmLpKeyInT_s : Inport  Port=15
  KBCM_RmLpKeyMissT_s : Inport  Port=16
  AND{,1..4} (5 alike) : Logic  AllPortsSameDT=off  OutDataTypeStr=boolean
  Chart : Stateflow chart  TreatAsAtomicUnit=on
      settings: PortSchema="{\"entries\":[{\"content\":{\"sides\":[{\"content\":{\"connectorIds\":[\"In1\",\"In2\",\"In3\",\"In4\",\"In5\",\"In6\",\"In7\",\"In10\",\"In11\",\"In12\",\"In13\",\"In9\",\"In8\"]},\"type\":\"ConnectorPlacement.EquallySpacedRectSide\",\"uuid\":\"6d4ef6e4-d310-4573-8670-c3ce7ffc5586\"},{\"content\":{\"connectorIds\":[\"Out1\",\"Out2\",\"Out3\"],\"side\":\"RIGHT\"},\"type\":\"ConnectorPlacement.EquallySpacedRectSide\",\"uuid\":\"4b29c1e1-9016-4f15-a64e-722acfc91947\"},{\"content\":{\"connectorIds\":[],\"side\":\"TOP\"},\"type\":\"ConnectorPlacement.EquallySpacedRectSide\",\"uuid\":\"c4982b23-9105-4f8b-8d41-99f0f59e85fc\"}]},\"type\":\"ConnectorPlacement.EquallySpacedConnector\",\"uuid\":\"68c6e652-9227-465e-b41e-a009e64da19a\"}],\"packageUris\":[\"http://schema.mathworks.com/mf0/Connector/R2020b\"],\"version\":\"1.0\"}"
  Constant{,1..4} (5 alike) : Constant  OutDataTypeStr=uint8
  Detect Increase{,1..4} (5 alike) : simulink/Logic and Bit Operations/Detect Increase  vinit=0.0  OutDataTypeStr=boolean
  Divide : Product  Inputs=*/
  Gain : Gain  Gain=MIN2SEC
  OR : Logic  Operator=OR  Inputs=5  AllPortsSameDT=off  OutDataTypeStr=boolean
  Terminator : Terminator
  Unit Delay{1..5} (5 alike) : UnitDelay  SampleTime=-1  HasFrameUpgradeWarning=on
  VBCM_RoomLampH_flg : Outport
  VBCM_RoomLampL_flg : Outport  Port=2
  wires:
  VBCM_BCMDoorLockSta_flg/1 -> Chart/3(DrLockSW)
  Chart/2(RoomLampL) -> VBCM_RoomLampL_flg/1  "VBCM_RoomLampL_flg"
  VPMM_PwrSta_enum/1 -> Chart/2(PwrSta)
  VBCM_AllDoorSW_flg/1 -> Chart/4(AllDoorSW)
  Chart/1(RoomLampH) -> VBCM_RoomLampH_flg/1  "VBCM_RoomLampH_flg"
  VBCM_AntitheftSta_enum/1 -> Chart/6(AntitheftSta)
  KBCM_RmLampKeep_min/1 -> Gain/1
  Gain/1 -> Divide/1
  FDC_BCM_RmLpModeENFun_Sta/1 -> Chart/9(FDC_BCM_RmLpModeENFun_Sta)
  Constant/1 -> Unit Delay1/1
  Unit Delay1/1 -> AND/1
  Detect Increase/1 -> AND/2
  VINP_DrDoorSW_flg/1 -> Detect Increase/1
  VINP_PsDoorSW_flg/1 -> Detect Increase1/1
  Detect Increase1/1 -> AND1/2
  Unit Delay2/1 -> AND1/1
  Constant1/1 -> Unit Delay2/1
  Constant2/1 -> Unit Delay3/1
  Unit Delay3/1 -> AND2/1
  Detect Increase2/1 -> AND2/2
  VINP_RLDoorSW_flg/1 -> Detect Increase2/1
  VINP_RRDoorSW_flg/1 -> Detect Increase3/1
  Detect Increase3/1 -> AND3/2
  Unit Delay4/1 -> AND3/1
  Constant3/1 -> Unit Delay4/1
  Constant4/1 -> Unit Delay5/1
  Unit Delay5/1 -> AND4/1
  Detect Increase4/1 -> AND4/2
  [VINP_TailgateSW_flg] -> Detect Increase4/1
  VINP_TailgateSW_flg/1 -> [VINP_TailgateSW_flg]
  [VINP_TailgateSW_flg] -> Chart/7(TailgateSW)
  AND/1 -> OR/1
  AND1/1 -> OR/2
  AND2/1 -> OR/3
  AND3/1 -> OR/4
  AND4/1 -> OR/5
  OR/1 -> [VBCM_DoorOpen_flg]
  [VBCM_DoorOpen_flg] -> Chart/5(DoorOpen)
  VINP_PDKeyAreaLockUnlock_enum/1 -> Chart/10(P_DKey_Area_LockUnlock)
  VINP_PDKeyAreaPS_enum/1 -> Chart/11(P_DKey_Area_PS)
  Chart/3(RoomLampTmr) -> Terminator/1  "VBCM_RoomLampTmr_s"
  KBCM_RmLpKeyInT_s/1 -> Chart/12(KBCM_RmLpKeyInT_s)  "2400"
  KBCM_RmLpKeyMissT_s/1 -> Chart/13(KBCM_RmLpKeyMissT_s)  "600"
  [task_time_s] -> Divide/2
  Divide/1 -> Chart/8(KBCM_RmLampKeep_min)
  task_time_s/1 -> [task_time_s]
  [task_time_s] -> Chart/1(task_time_s)

== system bcm/BCM/BCM/Tailgate ==
  VPMM_PwrSta_enum : Inport
  VINP_VehSpeed_kph : Inport  Port=2
  VBCM_BCMDoorLockSta_flg : Inport  Port=3
  VINP_TrunkHandleSwSG08_flg : Inport  Port=4
  VTQD_ShiftGearPosn_enum : Inport  Port=5
  Chart : Stateflow chart  TreatAsAtomicUnit=on
  VBCM_TrunkRel_flg : Outport
  VBCM_TailgateHDSW_flg : Outport  Port=2
  wires:
  VINP_VehSpeed_kph/1 -> Chart/2(VehSpeed)
  VBCM_BCMDoorLockSta_flg/1 -> Chart/3(DrLockSta)
  VINP_TrunkHandleSwSG08_flg/1 -> VBCM_TailgateHDSW_flg/1, Chart/5(TrunkHanSW)  "VBCM_TailgateHDSW_flg"
  Chart/1(TrunkRelease) -> VBCM_TrunkRel_flg/1  "VBCM_TrunkRel_flg"
  VPMM_PwrSta_enum/1 -> Chart/1(PwrSta)
  VTQD_ShiftGearPosn_enum/1 -> Chart/4(VTQD_ShiftGearPosn_enum)

== system bcm/BCM/BCM/Vehicle Type Diff Fun ==
  VINP_VehicleType_enum : Inport
  VINP_WlcmLightMode_enum : Inport  Port=2
  VPMM_PwrSta_enum : Inport  Port=3
  AND : Logic  AllPortsSameDT=off  OutDataTypeStr=boolean
  AND1 : Logic  Operator=OR  AllPortsSameDT=off  OutDataTypeStr=boolean
  AND2 : Logic  AllPortsSameDT=off  OutDataTypeStr=boolean
  Compare To Constant : simulink/Logic and Bit Operations/Compare To Constant  relop===  const=1  OutDataTypeStr=boolean
  Constant : Constant  Value=3
  Constant1 : Constant  Value=KBCM_RightHandDriveEN_flg
  Constant{2,5,7,10} (4 alike) : Constant  Value=ENUM_VEHICLETYPE_D31L24
  Constant3 : Constant  Value=4
  Constant4 : Constant  Value=TRUE
  Constant6 : Constant  Value=FALSE
  Constant8 : Constant  Value=ENUM_VEHICLETYPE_D21
  Constant9 : Constant  Value=ENUM_PWRSTASW_ON
  Data Type Conversion : DataTypeConversion  OutDataTypeStr=uint8
  Data Type Conversion1 : DataTypeConversion  OutDataTypeStr=uint8
  Equal{1..3,5} (4 alike) : RelationalOperator  Operator===  OutDataTypeStr=boolean  RndMeth=Simplest
  Equal4 : RelationalOperator  Operator=~=  OutDataTypeStr=boolean  RndMeth=Simplest
  Equal6 : RelationalOperator  Operator=<  OutDataTypeStr=boolean  RndMeth=Simplest
  Switch : Switch  Criteria=u2 > Threshold
  Switch1 : Switch  Criteria=u2 > Threshold
  VBCM_APMDoorCtrlEN_flg : Outport
  VBCM_RightHandDriveEN_flg : Outport  Port=2
  VBCM_HLBeamENPwrSta_enum : Outport  Port=3
  VBCM_showupEN_flg : Outport  Port=4
  VBCM_UnlockWelcomeEN_flg : Outport  Port=5
  wires:
  [VINP_VehicleType_enum] -> Equal3/1
  Constant10/1 -> Equal3/2
  VINP_VehicleType_enum/1 -> [VINP_VehicleType_enum]
  Equal3/1 -> VBCM_APMDoorCtrlEN_flg/1
  Constant1/1 -> VBCM_RightHandDriveEN_flg/1
  Constant2/1 -> Equal1/2
  [VINP_VehicleType_enum] -> Equal1/1
  Equal1/1 -> Switch/2
  Constant/1 -> Data Type Conversion/1
  Data Type Conversion/1 -> Switch/1
  Constant3/1 -> Data Type Conversion1/1
  Data Type Conversion1/1 -> Switch/3
  Switch/1 -> VBCM_HLBeamENPwrSta_enum/1
  Constant6/1 -> Switch1/3
  Constant4/1 -> Switch1/1
  Equal2/1 -> Switch1/2
  [VINP_VehicleType_enum] -> Equal2/1
  Constant5/1 -> Equal2/2
  Switch1/1 -> VBCM_showupEN_flg/1
  VINP_WlcmLightMode_enum/1 -> Compare To Constant/1
  Constant7/1 -> Equal4/2
  [VINP_VehicleType_enum] -> Equal4/1
  Equal4/1 -> AND/2
  Compare To Constant/1 -> AND/1
  AND/1 -> AND1/1
  [VINP_VehicleType_enum] -> Equal5/1
  Constant8/1 -> Equal5/2
  Equal5/1 -> AND1/2
  AND1/1 -> AND2/1
  Equal6/1 -> AND2/2
  VPMM_PwrSta_enum/1 -> Equal6/1
  Constant9/1 -> Equal6/2
  AND2/1 -> VBCM_UnlockWelcomeEN_flg/1

== system bcm/BCM/BCM/Verify ==
  VINP_FlashAntitheft_enum : Inport
  Constant1 : Constant  Value=ENUM_ANTITHEFT_DISARM
  Constant10 : Constant  Value=ENUM_ANTITHEFT_WAIT
  Constant11 : Constant  Value=ENUM_ANTITHEFT_ALARM
  Constant9 : Constant  Value=ENUM_ANTITHEFT_ARM
  Equal1 : RelationalOperator  Operator=~=  OutDataTypeStr=boolean  RndMeth=Simplest
  Equal2 : RelationalOperator  Operator=~=  OutDataTypeStr=boolean  RndMeth=Simplest
  Equal3 : RelationalOperator  Operator=~=  OutDataTypeStr=boolean  RndMeth=Simplest
  Logical Operator : Logic  Inputs=3  AllPortsSameDT=off  OutDataTypeStr=boolean
  Switch : Switch  Criteria=u2 > Threshold
  VBCM_FlashAntitheft_enum : Outport
  wires:
  Constant9/1 -> Equal1/2
  VINP_FlashAntitheft_enum/1 -> [VINP_FlashAntitheft_enum]
  [VINP_FlashAntitheft_enum] -> Equal2/1
  [VINP_FlashAntitheft_enum] -> Equal1/1
  Constant11/1 -> Equal3/2
  Constant10/1 -> Equal2/2
  [VINP_FlashAntitheft_enum] -> Equal3/1
  Switch/1 -> VBCM_FlashAntitheft_enum/1
  Logical Operator/1 -> Switch/2
  Constant1/1 -> Switch/1
  [VINP_FlashAntitheft_enum] -> Switch/3
  Equal1/1 -> Logical Operator/1
  Equal2/1 -> Logical Operator/2
  Equal3/1 -> Logical Operator/3

== system bcm/BCM/BCM/WasherWiper ==
  task_time_s : Inport
  VINP_CSWFWasSWSta_enum : Inport  Port=2
  VINP_CSWFWipSWSta_enum : Inport  Port=3
  VINP_RLSRainSnrWiperCmd_enum : Inport  Port=4
  VINP_FWiperAS_flg : Inport  Port=5
  VINP_CSWRWipIntSwSta_enum : Inport  Port=6
  VINP_RWiperAS_flg : Inport  Port=7
  VINP_CSWRWasSWSta_enum : Inport  Port=8
  VPMM_PwrSta_enum : Inport  Port=9
  VINP_IVIWIMAINSW_flg : Inport  Port=10
  VINP_CANMsgValidIVI2_flg : Inport  Port=11
  VINP_RWiperProtection_flg : Inport  Port=12
  VINP_FWiperProtection_flg : Inport  Port=13
  VINP_FlashWiperFixMode : Inport  Port=14
  BCMInitial : Inport  Port=15
  VINP_DiagWipRLSCmdCutEN_flg : Inport  Port=16
  VINP_DiagRLSCmdCutTime_s : Inport  Port=17
  VINP_DiagWipRLSCmdHoldEN_flg : Inport  Port=18
  VINP_DiagRLSCmdHoldTime_s : Inport  Port=19
  VINP_FlashAutoWipHSpdEN_flg : Inport  Port=20
  VINP_IVIAutoWipHSpdSWCmd_flg : Inport  Port=21
  VINP_IVICarWashModeCmd_flg : Inport  Port=22
  Chart : Stateflow chart  TreatAsAtomicUnit=on
      settings: PortSchema="{\"entries\":[{\"content\":{\"sides\":[{\"content\":{\"connectorIds\":[\"In1\",\"In2\",\"In12\",\"In4\",\"In5\",\"In3\",\"In6\",\"In7\",\"In8\",\"In9\",\"In10\",\"In11\",\"In14\",\"In13\"]},\"type\":\"ConnectorPlacement.EquallySpacedRectSide\",\"uuid\":\"ddf23117-5dc2-4a3f-b10f-289355e47226\"},{\"content\":{\"connectorIds\":[\"Out1\",\"Out2\",\"Out3\",\"Out4\"],\"side\":\"RIGHT\"},\"type\":\"ConnectorPlacement.EquallySpacedRectSide\",\"uuid\":\"3bf6cfe7-a7e6-42ff-b7c9-2b0f0784fdda\"},{\"content\":{\"connectorIds\":[],\"side\":\"TOP\"},\"type\":\"ConnectorPlacement.EquallySpacedRectSide\",\"uuid\":\"e8c554c5-f3ab-4c94-9a33-c4a286390113\"}]},\"type\":\"ConnectorPlacement.EquallySpacedConnector\",\"uuid\":\"1150097c-92a6-43a0-8ded-0f00109e7741\"}],\"packageUris\":[\"http://schema.mathworks.com/mf0/Connector/R2020b\"],\"version\":\"1.0\"}"
  Constant : Constant  Value=TRUE
  Data Type Conversion : DataTypeConversion  OutDataTypeStr=single
  Detect Increase : simulink/Logic and Bit Operations/Detect Increase  vinit=0.0  OutDataTypeStr=boolean
  Divide : Product  Inputs=*/
  NOT : Logic  Operator=NOT  AllPortsSameDT=off  OutDataTypeStr=boolean
  RLS_Command_Cut_Filter : Subsystem
  Saturation : Saturate  UpperLimit=9  LowerLimit=0
  Switch{,1..3} (4 alike) : Switch  Criteria=u2 > Threshold
  Unit Delay : UnitDelay  SampleTime=-1  HasFrameUpgradeWarning=on
  Unit Delay1 : UnitDelay  SampleTime=-1  HasFrameUpgradeWarning=on
  Unit Delay2 : UnitDelay  SampleTime=-1  HasFrameUpgradeWarning=on
  VBCM_FrWiperL_flg : Outport
  VBCM_FrWiperH_flg : Outport  Port=2
  VBCM_RrWiper_flg : Outport  Port=3
  VBCM_WasherCtrl_enum : Outport  Port=4
  VBCM_WiperFixMode_flg : Outport  Port=5
  VBCM_AutoWipHSpdENSta_flg : Outport  Port=6
  wires:
  Divide/1 -> Chart/14(DiagRLSCmdHoldTime)
  VINP_DiagWipRLSCmdHoldEN_flg/1 -> Chart/4(DiagWipRLSCmdHoldEN)
  [task_time_s] -> Divide/2
  VINP_DiagRLSCmdHoldTime_s/1 -> Data Type Conversion/1
  Data Type Conversion/1 -> Divide/1
  VINP_DiagRLSCmdCutTime_s/1 -> Saturation/1
  VINP_DiagWipRLSCmdCutEN_flg/1 -> RLS_Command_Cut_Filter/3(VINP_DiagWipRLSCmdCutEN_flg)
  [task_time_s] -> RLS_Command_Cut_Filter/2(task_time_s)
  task_time_s/1 -> [task_time_s]
  VINP_RLSRainSnrWiperCmd_enum/1 -> RLS_Command_Cut_Filter/1(VINP_RLSRainSnrWiperCmd_enum)
  RLS_Command_Cut_Filter/1(RLS_WiperCmd) -> Chart/12(RLS_WiperCmd)
  Switch/1 -> Switch1/1
  Switch1/1 -> Unit Delay/1, VBCM_WiperFixMode_flg/1  "VBCM_WiperFixMode_flg"
  VINP_FlashWiperFixMode/1 -> Switch1/3
  BCMInitial/1 -> Switch1/2
  Unit Delay/1 -> Switch/3
  VINP_CANMsgValidIVI2_flg/1 -> Switch/2
  VINP_IVIWIMAINSW_flg/1 -> Switch/1
  VINP_CSWRWipIntSwSta_enum/1 -> Chart/6(CSW_RWipIntSw_Sta)
  Chart/4(WasherControl) -> VBCM_WasherCtrl_enum/1  "VBCM_WasherCtrl_enum"
  Chart/3(RWiper) -> VBCM_RrWiper_flg/1  "VBCM_RrWiper_flg"
  VINP_CSWFWasSWSta_enum/1 -> Chart/1(CSW_FWasSw_Sta)
  VINP_CSWRWasSWSta_enum/1 -> Chart/8(CSW_RWasSW_Sta)
  VPMM_PwrSta_enum/1 -> Chart/9(PwrSta)
  VINP_CSWFWipSWSta_enum/1 -> Chart/2(CSW_FWipSw_Sta)
  VINP_FWiperAS_flg/1 -> Chart/3(FWiperAS)
  VINP_RWiperAS_flg/1 -> Chart/7(RWiperAS)
  Chart/2(FWiperH) -> VBCM_FrWiperH_flg/1  "VBCM_FrWiperH_flg"
  Chart/1(FWiperL) -> VBCM_FrWiperL_flg/1  "VBCM_FrWiperL_flg"
  VINP_RWiperProtection_flg/1 -> Chart/10(VINP_RWiperProtection_flg)
  VINP_FWiperProtection_flg/1 -> Chart/11(VINP_FWiperProtection_flg)
  Saturation/1 -> RLS_Command_Cut_Filter/4(VINP_DiagRLSCmdCutTime_s)
  Constant/1 -> Unit Delay1/1
  Unit Delay1/1 -> Switch2/2
  VINP_FlashAutoWipHSpdEN_flg/1 -> Switch2/3
  VINP_IVIAutoWipHSpdSWCmd_flg/1 -> Detect Increase/1
  Detect Increase/1 -> Switch3/2
  NOT/1 -> Switch3/1
  Switch3/1 -> Switch2/1
  Switch2/1 -> VBCM_AutoWipHSpdENSta_flg/1, Unit Delay2/1, [VBCM_AutoWipHSpdENSta_flg]
  Unit Delay2/1 -> NOT/1, Switch3/3
  [VBCM_AutoWipHSpdENSta_flg] -> Chart/5(FDC_BCM_AutoWipHSpdEN_Sta)
  VINP_IVICarWashModeCmd_flg/1 -> Chart/13(VINP_IVICarWashModeCmd_flg)

== system bcm/BCM/BCM/Window_Control_Sig_Combine ==
  VBCM_APMDoorCtrlEN_flg : Inport
  VBCM_RightHandDriveEN_flg : Inport  Port=2
  VINP_DKCDrvWdwCtrlCmd_pct : Inport  Port=3
  VINP_ConnDrvWdwCtrlCmd_pct : Inport  Port=4
  VBCM_BCMDrvWdwCtrlCmd_pct : Inport  Port=5
  VINP_LDrvControlCommand_pct : Inport  Port=6
  VINP_DKCPasWdwCtrlCmd_pct : Inport  Port=7
  VINP_ConnPasWdwCtrlCmd_pct : Inport  Port=8
  VBCM_BCMPasWdwCtrlCmd_pct : Inport  Port=9
  VINP_LPasControlCommand_pct : Inport  Port=10
  VINP_DKCRLDWdwCtrlCmd_pct : Inport  Port=11
  VINP_ConnRLDWdwCtrlCmd_pct : Inport  Port=12
  VBCM_BCMRLDWdwCtrlCmd_pct : Inport  Port=13
  VINP_LRLDControlCommand_pct : Inport  Port=14
  VINP_DKCRRDWdwCtrlCmd_pct : Inport  Port=15
  VINP_ConnRRDWdwCtrlCmd_pct : Inport  Port=16
  VBCM_BCMRRDWdwCtrlCmd_pct : Inport  Port=17
  VINP_LRRDControlCommand_pct : Inport  Port=18
  VINP_BDWinFOpenedSta_pct : Inport  Port=19
  VINP_BDWinROpenedSta_pct : Inport  Port=20
  VINP_BPWinFOpenedSta_pct : Inport  Port=21
  VINP_BPWinROpenedSta_pct : Inport  Port=22
  Constant{,1..3} (4 alike) : Constant  Value=127
  Data Type Conversion{,1..11} (12 alike) : DataTypeConversion  OutDataTypeStr=uint8
  Driver_Window : Subsystem
  Passenger_Window : Subsystem
  RearLeft_Window : Subsystem
  RearRight_Window : Subsystem
  Switch{,1..11} (12 alike) : Switch  Criteria=u2 > Threshold
  VBCM_DrvWdwCtrlCmd_pct : Outport
  VBCM_DrvWdwReqAP_enum : Outport  Port=2
  VBCM_PasWdwCtrlCmd_pct : Outport  Port=3
  VBCM_PasWdwReqAP_enum : Outport  Port=4
  VBCM_DrRWdwCtrlCmd_pct : Outport  Port=5
  VBCM_DrRWdwReqAP_enum : Outport  Port=6
  VBCM_PsRWdwCtrlCmd_pct : Outport  Port=7
  VBCM_PsRWdwReqAP_enum : Outport  Port=8
  VBCM_WinLFOpenedSta_pct : Outport  Port=9
  VBCM_WinRFOpenedSta_pct : Outport  Port=10
  VBCM_WinLROpenedSta_pct : Outport  Port=11
  VBCM_WinRROpenedSta_pct : Outport  Port=12
  wires:
  VINP_DKCDrvWdwCtrlCmd_pct/1 -> Driver_Window/1(DKCWINCMD)
  VINP_ConnDrvWdwCtrlCmd_pct/1 -> Driver_Window/3(CONNWINCMD)
  VBCM_BCMDrvWdwCtrlCmd_pct/1 -> Driver_Window/4(BCMWINCMD)
  Driver_Window/1(WINCMD) -> VBCM_DrvWdwCtrlCmd_pct/1
  Driver_Window/2(WINReqAP) -> VBCM_DrvWdwReqAP_enum/1
  Switch/1 -> Driver_Window/2(IVIWINCMD)
  Constant/1 -> Data Type Conversion/1
  Data Type Conversion/1 -> Switch/1
  VBCM_APMDoorCtrlEN_flg/1 -> [VBCM_APMDoorCtrlEN_flg]
  [VBCM_APMDoorCtrlEN_flg] -> Switch/2
  VINP_LDrvControlCommand_pct/1 -> Data Type Conversion4/1
  VINP_LPasControlCommand_pct/1 -> Data Type Conversion5/1
  [VBCM_APMDoorCtrlEN_flg] -> Switch1/2
  Data Type Conversion1/1 -> Switch1/1
  Constant1/1 -> Data Type Conversion1/1
  Switch1/1 -> Passenger_Window/2(IVIWINCMD)
  Switch2/1 -> RearLeft_Window/2(IVIWINCMD)
  Constant2/1 -> Data Type Conversion2/1
  Data Type Conversion2/1 -> Switch2/1
  [VBCM_APMDoorCtrlEN_flg] -> Switch2/2
  VINP_LRLDControlCommand_pct/1 -> Data Type Conversion6/1
  VINP_LRRDControlCommand_pct/1 -> Data Type Conversion7/1
  [VBCM_APMDoorCtrlEN_flg] -> Switch3/2
  Data Type Conversion3/1 -> Switch3/1
  Constant3/1 -> Data Type Conversion3/1
  VINP_DKCPasWdwCtrlCmd_pct/1 -> Passenger_Window/1(DKCWINCMD)
  VINP_ConnPasWdwCtrlCmd_pct/1 -> Passenger_Window/3(CONNWINCMD)
  VBCM_BCMPasWdwCtrlCmd_pct/1 -> Passenger_Window/4(BCMWINCMD)
  VINP_DKCRLDWdwCtrlCmd_pct/1 -> RearLeft_Window/1(DKCWINCMD)
  VINP_ConnRLDWdwCtrlCmd_pct/1 -> RearLeft_Window/3(CONNWINCMD)
  VBCM_BCMRLDWdwCtrlCmd_pct/1 -> RearLeft_Window/4(BCMWINCMD)
  VINP_DKCRRDWdwCtrlCmd_pct/1 -> RearRight_Window/1(DKCWINCMD)
  VINP_ConnRRDWdwCtrlCmd_pct/1 -> RearRight_Window/3(CONNWINCMD)
  VBCM_BCMRRDWdwCtrlCmd_pct/1 -> RearRight_Window/4(BCMWINCMD)
  Switch3/1 -> RearRight_Window/2(IVIWINCMD)
  Passenger_Window/1(WINCMD) -> VBCM_PasWdwCtrlCmd_pct/1
  Passenger_Window/2(WINReqAP) -> VBCM_PasWdwReqAP_enum/1
  RearLeft_Window/1(WINCMD) -> [VBCM_RLDWdwCtrlCmd_pct]
  RearLeft_Window/2(WINReqAP) -> [VBCM_RLDWdwReqAP_pct]
  RearRight_Window/1(WINCMD) -> [VBCM_RRDWdwCtrlCmd_pct]
  RearRight_Window/2(WINReqAP) -> [VBCM_RRDWdwReqAP_pct]
  VBCM_RightHandDriveEN_flg/1 -> [VBCM_RightHandDriveEN_flg]
  [VBCM_RightHandDriveEN_flg] -> Switch4/2
  Switch4/1 -> VBCM_DrRWdwCtrlCmd_pct/1
  [VBCM_RRDWdwCtrlCmd_pct] -> Switch4/1
  [VBCM_RLDWdwCtrlCmd_pct] -> Switch4/3
  [VBCM_RightHandDriveEN_flg] -> Switch5/2
  [VBCM_RLDWdwCtrlCmd_pct] -> Switch5/1
  [VBCM_RRDWdwCtrlCmd_pct] -> Switch5/3
  Switch5/1 -> VBCM_PsRWdwCtrlCmd_pct/1
  Switch6/1 -> VBCM_DrRWdwReqAP_enum/1
  Switch7/1 -> VBCM_PsRWdwReqAP_enum/1
  [VBCM_RightHandDriveEN_flg] -> Switch6/2
  [VBCM_RLDWdwReqAP_pct] -> Switch6/3
  [VBCM_RRDWdwReqAP_pct] -> Switch6/1
  [VBCM_RRDWdwReqAP_pct] -> Switch7/3
  [VBCM_RightHandDriveEN_flg] -> Switch7/2
  [VBCM_RLDWdwReqAP_pct] -> Switch7/1
  Data Type Conversion4/1 -> Switch/3
  Data Type Conversion5/1 -> Switch1/3
  Data Type Conversion6/1 -> Switch2/3
  Data Type Conversion7/1 -> Switch3/3
  [VBCM_RightHandDriveEN_flg] -> Switch8/2
  VINP_BPWinROpenedSta_pct/1 -> [VINP_BPWinROpenedSta_pct]
  VINP_BPWinFOpenedSta_pct/1 -> [VINP_BPWinFOpenedSta_pct]
  VINP_BDWinROpenedSta_pct/1 -> [VINP_BDWinROpenedSta_pct]
  VINP_BDWinFOpenedSta_pct/1 -> [VINP_BDWinFOpenedSta_pct]
  [VINP_BDWinFOpenedSta_pct] -> Switch8/3
  [VINP_BPWinFOpenedSta_pct] -> Switch8/1
  Switch8/1 -> Data Type Conversion8/1
  [VBCM_RightHandDriveEN_flg] -> Switch9/2
  [VBCM_RightHandDriveEN_flg] -> Switch10/2
  [VBCM_RightHandDriveEN_flg] -> Switch11/2
  [VINP_BDWinFOpenedSta_pct] -> Switch9/1
  [VINP_BPWinFOpenedSta_pct] -> Switch9/3
  Switch9/1 -> Data Type Conversion9/1
  Switch10/1 -> Data Type Conversion10/1
  Switch11/1 -> Data Type Conversion11/1
  [VINP_BDWinROpenedSta_pct] -> Switch10/3
  [VINP_BPWinROpenedSta_pct] -> Switch10/1
  [VINP_BPWinROpenedSta_pct] -> Switch11/3
  [VINP_BDWinROpenedSta_pct] -> Switch11/1
  Data Type Conversion8/1 -> VBCM_WinLFOpenedSta_pct/1
  Data Type Conversion9/1 -> VBCM_WinRFOpenedSta_pct/1
  Data Type Conversion10/1 -> VBCM_WinLROpenedSta_pct/1
  Data Type Conversion11/1 -> VBCM_WinRROpenedSta_pct/1

== system bcm/BCM/BCM/APM_Door/DoorAPM ==
  task_time_s : Inport
  DoorSW_flg : Inport  Port=2
  ControlCommand_pct : Inport  Port=3
  ValWdwOpened_pct : Inport  Port=4
  APMDoorControlSta_flg : Inport  Port=5
  WaitAPMPwr_K : Inport  Port=6
  DrOpenWdwOT_s : Inport  Port=7
  DrOpenWdwReady_s : Inport  Port=8
  KBCM_WdwManualDetT_K : Inport  Port=9
  CANMsgValidIVI2 : Inport  Port=10
  CANMsgValidGWZoneDR1 : Inport  Port=11
  CANMsgValidGWZoneFR1 : Inport  Port=12
  KBCM_DrAPMRetryTimes_cnt : Inport  Port=13
  VINP_CANMsgValidzGWLINDr1_flg : Inport  Port=14
  Compare To Constant12 : simulink/Logic and Bit Operations/Compare To Constant  relop=>=  const=126  OutDataTypeStr=boolean
  Constant : Constant  Value=127
  Data Type Conversion{,1,4,8} (4 alike) : DataTypeConversion  OutDataTypeStr=uint8
  Data Type Conversion2 : DataTypeConversion  OutDataTypeStr=boolean
  Divide : Product  Inputs=*/
  Divide1 : Product  Inputs=*/
  Equal : RelationalOperator  OutDataTypeStr=boolean  RndMeth=Simplest
  Logical Operator : Logic  Operator=NOT  AllPortsSameDT=off  OutDataTypeStr=boolean
  Switch : Switch  Criteria=u2 ~= 0
  Switch1 : Switch  Criteria=u2 > Threshold
  Timer : hcu_lib/Basic_Blocks/Timer
  Unit Delay : UnitDelay  SampleTime=-1  HasFrameUpgradeWarning=on
  Unit Delay9 : UnitDelay  SampleTime=-1  HasFrameUpgradeWarning=on
  window : Stateflow chart  TreatAsAtomicUnit=on
      settings: PortSchema="{\"entries\":[{\"content\":{\"sides\":[{\"content\":{\"connectorIds\":[\"In1\",\"In6\",\"In2\",\"In5\",\"In4\",\"In3\",\"In7\",\"In8\",\"In9\",\"In10\",\"In11\"]},\"type\":\"ConnectorPlacement.EquallySpacedRectSide\",\"uuid\":\"d6b3deb8-ac04-4a5e-8f43-f0925f49394b\"},{\"content\":{\"connectorIds\":[\"Out1\"],\"side\":\"RIGHT\"},\"type\":\"ConnectorPlacement.EquallySpacedRectSide\",\"uuid\":\"aa7d2074-5c17-49a8-96c4-41ae3a8edd6e\"},{\"content\":{\"side\":\"TOP\"},\"type\":\"ConnectorPlacement.EquallySpacedRectSide\",\"uuid\":\"a289e248-55db-4799-9cc5-9ff36bce4275\"}]},\"type\":\"ConnectorPlacement.EquallySpacedConnector\",\"uuid\":\"319072de-6de5-41b6-a853-dccc1445f214\"}],\"packageUris\":[\"http://schema.mathworks.com/mf0/Connector/R2020b\"],\"version\":\"1.0\"}"
  CtrlCmd_pct : Outport
  CtrlCmdReady_flg : Outport  Port=2
  wires:
  Data Type Conversion2/1 -> window/5(CtrlCmd_Ready)
  KBCM_DrAPMRetryTimes_cnt/1 -> window/11(KBCM_DrAPMRetryTimes_cnt)
  CANMsgValidGWZoneFR1/1 -> window/10(CANMsgValidGWZoneFR1)
  CANMsgValidGWZoneDR1/1 -> window/9(CANMsgValidGWZoneDR1)
  ControlCommand_pct/1 -> Switch/1
  Unit Delay/1 -> Switch/3
  Switch/1 -> Unit Delay/1, Data Type Conversion8/1
  CANMsgValidIVI2/1 -> Switch/2
  Divide1/1 -> Data Type Conversion1/1
  Data Type Conversion1/1 -> window/8(KBCM_WdwManualDetT_K)
  KBCM_WdwManualDetT_K/1 -> Divide1/1
  [task_time_s] -> Divide1/2
  [DrOpenWdwReady_s] -> Equal/2
  [DrOpenWdwReady_s] -> Timer/4
  DrOpenWdwReady_s/1 -> [DrOpenWdwReady_s]
  DrOpenWdwOT_s/1 -> Divide/1
  [task_time_s] -> Divide/2
  Divide/1 -> Data Type Conversion4/1
  WaitAPMPwr_K/1 -> window/3(WaitAPMPwr_K)
  APMDoorControlSta_flg/1 -> window/4(APMDoorControlSta)
  task_time_s/1 -> [task_time_s]
  Unit Delay9/1 -> Data Type Conversion2/1
  [task_time_s] -> Timer/3
  [CtrlCmdReady_flg] -> Unit Delay9/1
  Logical Operator/1 -> Timer/2
  Data Type Conversion/1 -> window/2(Val_Wdw_Opened)
  DoorSW_flg/1 -> window/1(DoorSW)
  Data Type Conversion4/1 -> window/7(DrOpenWdwOT_K)
  Compare To Constant12/1 -> Timer/1, Logical Operator/1
  window/1(CtrlCmd) -> CtrlCmd_pct/1, Compare To Constant12/1
  Timer/1 -> Equal/1
  Data Type Conversion8/1 -> window/6(ControlCommand)
  Equal/1 -> [CtrlCmdReady_flg], CtrlCmdReady_flg/1
  VINP_CANMsgValidzGWLINDr1_flg/1 -> Switch1/2
  Constant/1 -> Switch1/3
  Switch1/1 -> Data Type Conversion/1
  ValWdwOpened_pct/1 -> Switch1/1

== system bcm/BCM/BCM/AntiTheft/Antitheft__override ==
  In1 : Inport
  Constant : Constant  Value=KBCM_Antitheft_enum_ovrdflg
  Constant1 : Constant  Value=KBCM_Antitheft_enum_ovrdval
  Switch : Switch  Criteria=u2 > Threshold
  Out1 : Outport
  wires:
  Constant/1 -> Switch/2
  Switch/1 -> Out1/1
  In1/1 -> Switch/3
  Constant1/1 -> Switch/1

== system bcm/BCM/BCM/ExteriorLight/HeadLampErrorHanding ==
  VINP_HeadLampSW_enum : Inport
  VINP_CANMsgValidIVI2_flg : Inport  Port=2
  Add : Sum
  Compare To Constant : simulink/Logic and Bit Operations/Compare To Constant  relop=>=  const=1000  OutDataTypeStr=boolean
  Constant : Constant
  Constant1 : Constant  Value=0
  Constant2 : Constant  Value=0
  Constant3 : Constant  Value=0
  Saturation : Saturate  UpperLimit=1000  LowerLimit=0
  Switch{,1..3} (4 alike) : Switch  Criteria=u2 > Threshold
  Unit Delay : UnitDelay  SampleTime=-1  HasFrameUpgradeWarning=on
  Unit Delay1 : UnitDelay  SampleTime=-1  HasFrameUpgradeWarning=on
  VBCM_HeadLampSW_enum : Outport
  wires:
  VINP_CANMsgValidIVI2_flg/1 -> Switch2/2, Switch/2
  Switch2/1 -> Switch3/3, Unit Delay/1
  Unit Delay/1 -> Switch2/3
  VINP_HeadLampSW_enum/1 -> Switch2/1
  Switch/1 -> Switch1/2, Add/2
  Unit Delay1/1 -> Add/1
  Add/1 -> Switch1/1
  Constant/1 -> Switch/3
  Constant1/1 -> Switch/1
  Constant2/1 -> Switch1/3
  Constant3/1 -> Switch3/1
  Switch3/1 -> VBCM_HeadLampSW_enum/1
  Compare To Constant/1 -> Switch3/2
  Saturation/1 -> Unit Delay1/1, Compare To Constant/1
  Switch1/1 -> Saturation/1

== system bcm/BCM/BCM/HMI_Custom_Button/Key1 ==
  KeyNum : Inport
  IVI_HMICustmKEY_Sta : Inport  Port=2
  IVI_HMICustmFun_Sta : Inport  Port=3
  KeyFuncMem : Inport  Port=4
  PreSetFunc : Inport  Port=5
  InitialBar : Inport  Port=6
  Data Type Conversion : DataTypeConversion  OutDataTypeStr=uint8
  Equal : RelationalOperator  Operator===  OutDataTypeStr=boolean  RndMeth=Simplest
  Switch : Switch  Criteria=u2 > Threshold
  Switch1 : Switch  Criteria=u2 > Threshold
  Switch2 : Switch  Criteria=u2 > Threshold
  Unit Delay : UnitDelay  SampleTime=-1  HasFrameUpgradeWarning=on
  KeyFunc : Outport
  wires:
  IVI_HMICustmKEY_Sta/1 -> Equal/2
  Equal/1 -> Switch/2
  IVI_HMICustmFun_Sta/1 -> Switch/1
  KeyFuncMem/1 -> Switch1/2, Switch1/1
  PreSetFunc/1 -> Switch1/3
  Switch1/1 -> Switch2/3
  InitialBar/1 -> Switch2/2
  Switch2/1 -> Unit Delay/1, KeyFunc/1
  Switch/1 -> Switch2/1
  Unit Delay/1 -> Switch/3
  KeyNum/1 -> Data Type Conversion/1
  Data Type Conversion/1 -> Equal/1
